simulink model "SysModelLQR"  (R2018a)
settings: Solver=VariableStepAuto  StartTime=0.0  StopTime=6.0  RelTol=1e-3
values from neighbouring files (symbols this model uses):
  A = [0      1              0           0 ... (first row only)    [PendulumSSModel.m]    (also in PendulumSSModel_LQR.m = [0                 1                 0                 0; PendulumSSModel_Metric.m = [0                 1                 0                 0; PendulumSSModel_Metric_fxn.m = [0                 1                 0                 0)
  B = [     0 ... (first row only)    [PendulumSSModel.m]    (also in PendulumSSModel_LQR.m = [        0; PendulumSSModel_Metric.m; PendulumSSModel_Metric_fxn.m)
  K = lqr(A,B,Q,R)    [PendulumSSModel_LQR.m]
settings Model: Creator=jcl54  LastModifiedBy=bmo6

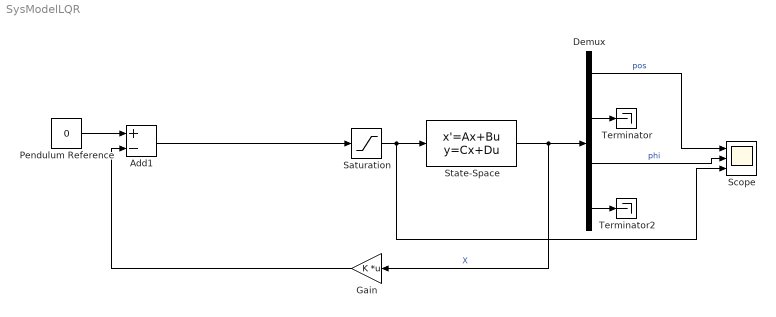
== system SysModelLQR ==
  Add1 : Sum  Inputs=+-
  Demux : Demux
  Gain : Gain  Gain=K  Multiplication=Matrix(K*u)
  Pendulum Reference : Constant  Value=0
  Saturation : Saturate  UpperLimit=3.8  LowerLimit=-3.8
  Scope : Scope  NumInputPorts=3
  State-Space : StateSpace  A=A  B=B  C=eye(4)  D=zeros(4,1)  InitialCondition=[0,0,0.075,0]  ContinuousStateAttributes={'x','x_dot','phi','phi_dot'}
  Terminator : Terminator
  Terminator2 : Terminator
  wires:
  Pendulum Reference/1 -> Add1/1
  Add1/1 -> Saturation/1
  State-Space/1 -> Gain/1, Demux/1  "X"
  Demux/2 -> Terminator/1
  Demux/3 -> Scope/2  "phi"
  Demux/4 -> Terminator2/1
  Demux/1 -> Scope/1  "pos"
  Saturation/1 -> Scope/3, State-Space/1
  Gain/1 -> Add1/2
